simulink model "Appl_VentAdj_CtrlModel"  (R2018b)
settings: configuration reference "CodeConfig_10_ms" (kept outside this file)
undefined symbols (not defined in the file): D_VENT_LVL_1_PRECENT, D_VENT_LVL_2_PRECENT, D_VENT_LVL_3_PRECENT, FALSE, TRUE
libraries: DareLib x72, simulink x1
(part 4 of 4)

== stateflow chart Appl_VentAdj_CtrlModel/LogicCtrl/LocalAdjustCtrl/VentLevelDeal/LevelAquireFunction4/LevelAquireFunction ==
  state LevelAquire
    (default) -> (junction 92)
    LevelAquire -> (junction 92)
    (junction 92) -> (junction 95) [order 1] : /*加热功能禁能
        | || OFF 电
        | || 发动机不在运行中*/
        | [enVentStopReason.EN_VENT_STOP_R_NONE != DisableSts ...
        | || FALSE == EnableCfg ...
        | || enPowerModeSts.EN_OFF == PowerMode ...
        | || TRUE != EngineSts]
    (junction 92) -> (junction 94) [order 2] : {StopFlag = FALSE;}
    (junction 95) -> (junction 93) : {Level = enVentLvlSts.EN_VENT_LVL_OFF;
        | StopFlag = TRUE;}
    (junction 93) -> (junction 94)
    (junction 94) -> (junction 101)
    (junction 101) -> (junction 21) [order 1] : [StopFlag == FALSE]
    (junction 21) -> (junction 23) [order 1] : [enProjectType.EN_PROJECT_P20 == CarTypeCfg]
    (junction 101) -> (junction 104) [order 2] : {Level = enVentLvlSts.EN_VENT_LVL_OFF;}
    (junction 21) -> (junction 48) [order 2]
    (junction 23) -> (junction 82)
    (junction 82) -> (junction 84) [order 1] : /* 一键开启 且为Hmi控制 */
        | [5 == CAN_Message && Type == 0]
    (junction 82) -> (junction 25) [order 2]
    (junction 84) -> (junction 86) : {Level = CAN_Lvl + 1;}
    (junction 25) -> (junction 27) [order 1] : [4 == CAN_Message]
    (junction 25) -> (junction 29) [order 2] : {TempMsg = CAN_Message + 7;}
    (junction 27) -> (junction 57) : {Level = enVentLvlSts.EN_VENT_LVL_OFF;}
    (junction 48) -> (junction 50) [order 1] : [1 != CAN_Message]
    (junction 48) -> (junction 55) [order 2] : {Level = enVentLvlSts.EN_VENT_LVL_OFF;}
    (junction 50) -> (junction 52) : {TempMsg = CAN_Message;}
    (junction 52) -> (junction 29)
    (junction 29) -> (junction 32) [order 1] : [7 < TempMsg && 11 > TempMsg]
    (junction 29) -> (junction 36) [order 2] : {Level = 0xFF;}
    (junction 32) -> (junction 34)
    (junction 34) -> (junction 38) [order 1] : [8 == TempMsg]
    (junction 34) -> (junction 40) [order 2]
    (junction 38) -> (junction 59) : {Level = enVentLvlSts.EN_VENT_LVL_1;}
    (junction 40) -> (junction 42) [order 1] : [9 == TempMsg]
    (junction 40) -> (junction 46) [order 2] : {Level = enVentLvlSts.EN_VENT_LVL_3;}
    (junction 42) -> (junction 44) : {Level = enVentLvlSts.EN_VENT_LVL_2;}
    (junction 55) -> (junction 104)
    (junction 36) -> (junction 55)
    (junction 46) -> (junction 36)
    (junction 44) -> (junction 46)
    (junction 59) -> (junction 44)
    (junction 57) -> (junction 59)
    (junction 86) -> (junction 57)
    (junction 104) -> (junction 75)
  data: EnableCfg input uint8; CarTypeCfg input Enum: enProjectType; PowerMode input Enum: enPowerModeSts; EngineSts input uint8; CAN_Message input uint8; DisableSts input Enum: enVentStopReason; Level output uint8; TempMsg local uint8; TRUE parameter; FALSE parameter; CAN_Lvl input uint8; Type input; StopFlag local boolean

== stateflow chart Appl_VentAdj_CtrlModel/UpDataInputInfo/InputSignalProcess/VentMessage/VentMessage/MsgConflictFunction2/Function ==
  state HMI_MessageDeal [parallel]
    settings: executionOrder=1
    state Default
      en:
      HMI_Flag = FALSE;
    state Valid
      en:
      HMI_Flag = TRUE;
    (default) -> HMI_MessageDeal.Default
    HMI_MessageDeal.Default -> HMI_MessageDeal.Valid : /*HMI通风报文有效0x0:Inactive；0x1:Level 1；1档;0x2:Level 2；2档;0x3:Level 3；3档；0x4:OFF: 0x05 OPEN*/
        | [enVentLvlSts.EN_VENT_LVL_1 == HMI_Message ...
        | || enVentLvlSts.EN_VENT_LVL_2 == HMI_Message ...
        | || enVentLvlSts.EN_VENT_LVL_3 == HMI_Message ...
        | || 4 == HMI_Message || 5 == HMI_Message]
    HMI_MessageDeal.Valid -> HMI_MessageDeal.Default : /*HMI通风报文无效，20240507NXM增加关闭4*/
        | [enVentLvlSts.EN_VENT_LVL_1 != HMI_Message ...
        | && enVentLvlSts.EN_VENT_LVL_2 != HMI_Message ...
        | && enVentLvlSts.EN_VENT_LVL_3 != HMI_Message ...
        | && 4 != HMI_Message && 5 != HMI_Message]
  state Tbox_MessageDeal [parallel]
    settings: executionOrder=2
    state Default
      en:
      Tbox_Flag = FALSE;
    state Valid
      en:
      Tbox_Flag = TRUE;
    (default) -> Tbox_MessageDeal.Default
    Tbox_MessageDeal.Default -> Tbox_MessageDeal.Valid : /*Tbox通风报文有效0x0:No Request；0x1:Heat_1；0x2:Heat_2；0x3:Heat_3；0x4:Close*/
        | [enVentLvlSts.EN_VENT_LVL_1 == Tbox_Message ...
        | || enVentLvlSts.EN_VENT_LVL_2 == Tbox_Message ...
        | || enVentLvlSts.EN_VENT_LVL_3 == Tbox_Message ...
        | || 4 == Tbox_Message]
    Tbox_MessageDeal.Valid -> Tbox_MessageDeal.Default : /*Tbox通风报文无效，20240507NXM增加关闭4*/
        | [enVentLvlSts.EN_VENT_LVL_1 != Tbox_Message ...
        | && enVentLvlSts.EN_VENT_LVL_2 != Tbox_Message ...
        | && enVentLvlSts.EN_VENT_LVL_3 != Tbox_Message ...
        | && 4 != Tbox_Message]
  state MessageConflictDeal [parallel]
    settings: executionOrder=3
    state Default
      en,du:
      OutMsgHMI = HMI_Message;
      OutMsgTbox = Tbox_Message;
      MixConflictFlg = FALSE;
    state VentilateConflict
      en:
      OutMsgHMI = 0;
      OutMsgTbox = 0;
      MixConflictFlg = TRUE;
    state HeatConflict
      en:
      OutMsgHMI = 0;
      OutMsgTbox = 0;
      MixConflictFlg = FALSE;
    (default) -> MessageConflictDeal.Default
    MessageConflictDeal.Default -> VentilateConflict [order 2] : /*通风加热报文同时有效 且非关闭状态 */
        | [FALSE != VentValidFlag ...
        | && ((FALSE != HMI_Flag && 4 != HMI_Message) ...
        | || (FALSE != Tbox_Flag && 4 != Tbox_Message))]
    VentilateConflict -> MessageConflictDeal.Default [order 2] : /*通风加热报文不同时有效 或关闭，20240507NXM修改跳转顺序*/
        | [FALSE == VentValidFlag ...
        | || 4 == HMI_Message ...
        | || 4 == Tbox_Message]
    MessageConflictDeal.Default -> HeatConflict [order 1] : /*P20车型HMI、TBOX通风报文同时有效*/
        | [enProjectType.EN_PROJECT_P20 == CarTypeCfg ...
        | && FALSE != HMI_Flag ...
        | && FALSE != Tbox_Flag]
    HeatConflict -> MessageConflictDeal.Default [order 2] : /*非P20车型||P20车型通风报文不同时有效，20240507NXM*/
        | [enProjectType.EN_PROJECT_P20 != CarTypeCfg ...
        | || (enProjectType.EN_PROJECT_P20 == CarTypeCfg ...
        | && (FALSE == HMI_Flag || FALSE == Tbox_Flag))]
    VentilateConflict -> HeatConflict [order 1] : /*P20车型HMI、TBOX通风报文同时有效*/
        | [enProjectType.EN_PROJECT_P20 == CarTypeCfg ...
        | && FALSE != HMI_Flag ...
        | && FALSE != Tbox_Flag ...
        | && FALSE == VentValidFlag]
    HeatConflict -> VentilateConflict [order 1] : /*通风加热报文同时有效，20240507NXM*/
        | [FALSE != VentValidFlag ...
        | && (FALSE != HMI_Flag ...
        | || FALSE != Tbox_Flag)]
  data: CarTypeCfg input uint8; HMI_Message input; Tbox_Message input; VentValidFlag input uint8; FALSE parameter; OutMsgHMI output uint8; OutMsgTbox output uint8; HMI_Flag local uint8; Tbox_Flag local uint8; TRUE parameter; MixConflictFlg output uint8

== stateflow chart Appl_VentAdj_CtrlModel/LogicCtrl/LocalAdjustCtrl/VentLevelDeal/LevelAquireFunction5/LevelAquireFunction ==
  state LevelAquire
    (default) -> (junction 92)
    LevelAquire -> (junction 92)
    (junction 92) -> (junction 95) [order 1] : /*加热功能禁能
        | || OFF 电
        | || 发动机不在运行中*/
        | [enVentStopReason.EN_VENT_STOP_R_NONE != DisableSts ...
        | || FALSE == EnableCfg ...
        | || enPowerModeSts.EN_OFF == PowerMode ...
        | || TRUE != EngineSts]
    (junction 92) -> (junction 94) [order 2] : {StopFlag = FALSE;}
    (junction 95) -> (junction 93) : {Level = enVentLvlSts.EN_VENT_LVL_OFF;
        | StopFlag = TRUE;}
    (junction 93) -> (junction 94)
    (junction 94) -> (junction 101)
    (junction 101) -> (junction 21) [order 1] : [StopFlag == FALSE]
    (junction 21) -> (junction 23) [order 1] : [enProjectType.EN_PROJECT_P20 == CarTypeCfg]
    (junction 101) -> (junction 104) [order 2] : {Level = enVentLvlSts.EN_VENT_LVL_OFF;}
    (junction 21) -> (junction 48) [order 2]
    (junction 23) -> (junction 82)
    (junction 82) -> (junction 84) [order 1] : /* 一键开启 且为Hmi控制 */
        | [5 == CAN_Message && Type == 0]
    (junction 82) -> (junction 25) [order 2]
    (junction 84) -> (junction 86) : {Level = CAN_Lvl + 1;}
    (junction 25) -> (junction 27) [order 1] : [4 == CAN_Message]
    (junction 25) -> (junction 29) [order 2] : {TempMsg = CAN_Message + 7;}
    (junction 27) -> (junction 57) : {Level = enVentLvlSts.EN_VENT_LVL_OFF;}
    (junction 48) -> (junction 50) [order 1] : [1 != CAN_Message]
    (junction 48) -> (junction 55) [order 2] : {Level = enVentLvlSts.EN_VENT_LVL_OFF;}
    (junction 50) -> (junction 52) : {TempMsg = CAN_Message;}
    (junction 52) -> (junction 29)
    (junction 29) -> (junction 32) [order 1] : [7 < TempMsg && 11 > TempMsg]
    (junction 29) -> (junction 36) [order 2] : {Level = 0xFF;}
    (junction 32) -> (junction 34)
    (junction 34) -> (junction 38) [order 1] : [8 == TempMsg]
    (junction 34) -> (junction 40) [order 2]
    (junction 38) -> (junction 59) : {Level = enVentLvlSts.EN_VENT_LVL_1;}
    (junction 40) -> (junction 42) [order 1] : [9 == TempMsg]
    (junction 40) -> (junction 46) [order 2] : {Level = enVentLvlSts.EN_VENT_LVL_3;}
    (junction 42) -> (junction 44) : {Level = enVentLvlSts.EN_VENT_LVL_2;}
    (junction 55) -> (junction 104)
    (junction 36) -> (junction 55)
    (junction 46) -> (junction 36)
    (junction 44) -> (junction 46)
    (junction 59) -> (junction 44)
    (junction 57) -> (junction 59)
    (junction 86) -> (junction 57)
    (junction 104) -> (junction 75)
  data: EnableCfg input uint8; CarTypeCfg input Enum: enProjectType; PowerMode input Enum: enPowerModeSts; EngineSts input uint8; CAN_Message input uint8; DisableSts input Enum: enVentStopReason; Level output uint8; TempMsg local uint8; TRUE parameter; FALSE parameter; CAN_Lvl input uint8; Type input; StopFlag local boolean

== stateflow chart Appl_VentAdj_CtrlModel/UpDataInputInfo/InputSignalProcess/CommonPreconditionDeal/Deal ==
  state Default
    en:
    ComPCSatisfiedFlag = FALSE;
  state ValidSts
    en:
    ComPCSatisfiedFlag = TRUE;
  (default) -> Default
  Default -> ValidSts : /*(发动机运行中 || 整车运行状态满足) && 正常电压模式*/
      | [(TRUE == EngineRunningFlag || TRUE == VehicleRunFlag) ...
      | && enFinalPowerMode.EN_NORMAL_VOLT == VentAdj_VoltMode]
  ValidSts -> Default : /*(发动机不在运行中 && 整车运行状态不满足) || 非正常电压模式*/
      | [(TRUE != EngineRunningFlag && TRUE != VehicleRunFlag) ...
      | || enFinalPowerMode.EN_NORMAL_VOLT != VentAdj_VoltMode]
  data: EngineRunningFlag input; VehicleRunFlag input; ComPCSatisfiedFlag output uint8; TRUE parameter; FALSE parameter; VentAdj_VoltMode input

== stateflow chart Appl_VentAdj_CtrlModel/UpDataInputInfo/InputSignalProcess/VentMessage/VentMessage/MsgConflictFunction/Function ==
  state HMI_MessageDeal [parallel]
    settings: executionOrder=1
    state Default
      en:
      HMI_Flag = FALSE;
    state Valid
      en:
      HMI_Flag = TRUE;
    (default) -> HMI_MessageDeal.Default
    HMI_MessageDeal.Default -> HMI_MessageDeal.Valid : /*HMI通风报文有效0x0:Inactive；0x1:Level 1；1档;0x2:Level 2；2档;0x3:Level 3；3档；0x4:OFF: 0x05 OPEN*/
        | [enVentLvlSts.EN_VENT_LVL_1 == HMI_Message ...
        | || enVentLvlSts.EN_VENT_LVL_2 == HMI_Message ...
        | || enVentLvlSts.EN_VENT_LVL_3 == HMI_Message ...
        | || 4 == HMI_Message || 5 == HMI_Message]
    HMI_MessageDeal.Valid -> HMI_MessageDeal.Default : /*HMI通风报文无效，20240507NXM增加关闭4*/
        | [enVentLvlSts.EN_VENT_LVL_1 != HMI_Message ...
        | && enVentLvlSts.EN_VENT_LVL_2 != HMI_Message ...
        | && enVentLvlSts.EN_VENT_LVL_3 != HMI_Message ...
        | && 4 != HMI_Message && 5 != HMI_Message]
  state Tbox_MessageDeal [parallel]
    settings: executionOrder=2
    state Default
      en:
      Tbox_Flag = FALSE;
    state Valid
      en:
      Tbox_Flag = TRUE;
    (default) -> Tbox_MessageDeal.Default
    Tbox_MessageDeal.Default -> Tbox_MessageDeal.Valid : /*Tbox通风报文有效0x0:No Request；0x1:Heat_1；0x2:Heat_2；0x3:Heat_3；0x4:Close*/
        | [enVentLvlSts.EN_VENT_LVL_1 == Tbox_Message ...
        | || enVentLvlSts.EN_VENT_LVL_2 == Tbox_Message ...
        | || enVentLvlSts.EN_VENT_LVL_3 == Tbox_Message ...
        | || 4 == Tbox_Message]
    Tbox_MessageDeal.Valid -> Tbox_MessageDeal.Default : /*Tbox通风报文无效，20240507NXM增加关闭4*/
        | [enVentLvlSts.EN_VENT_LVL_1 != Tbox_Message ...
        | && enVentLvlSts.EN_VENT_LVL_2 != Tbox_Message ...
        | && enVentLvlSts.EN_VENT_LVL_3 != Tbox_Message ...
        | && 4 != Tbox_Message]
  state MessageConflictDeal [parallel]
    settings: executionOrder=3
    state Default
      en,du:
      OutMsgHMI = HMI_Message;
      OutMsgTbox = Tbox_Message;
      MixConflictFlg = FALSE;
    state VentilateConflict
      en:
      OutMsgHMI = 0;
      OutMsgTbox = 0;
      MixConflictFlg = TRUE;
    state HeatConflict
      en:
      OutMsgHMI = 0;
      OutMsgTbox = 0;
      MixConflictFlg = FALSE;
    (default) -> MessageConflictDeal.Default
    MessageConflictDeal.Default -> VentilateConflict [order 2] : /*通风加热报文同时有效 且非关闭状态 */
        | [FALSE != VentValidFlag ...
        | && ((FALSE != HMI_Flag && 4 != HMI_Message) ...
        | || (FALSE != Tbox_Flag && 4 != Tbox_Message))]
    VentilateConflict -> MessageConflictDeal.Default [order 2] : /*通风加热报文不同时有效 或关闭，20240507NXM修改跳转顺序*/
        | [FALSE == VentValidFlag ...
        | || 4 == HMI_Message ...
        | || 4 == Tbox_Message]
    MessageConflictDeal.Default -> HeatConflict [order 1] : /*P20车型HMI、TBOX通风报文同时有效*/
        | [enProjectType.EN_PROJECT_P20 == CarTypeCfg ...
        | && FALSE != HMI_Flag ...
        | && FALSE != Tbox_Flag]
    HeatConflict -> MessageConflictDeal.Default [order 2] : /*非P20车型||P20车型通风报文不同时有效，20240507NXM*/
        | [enProjectType.EN_PROJECT_P20 != CarTypeCfg ...
        | || (enProjectType.EN_PROJECT_P20 == CarTypeCfg ...
        | && (FALSE == HMI_Flag || FALSE == Tbox_Flag))]
    VentilateConflict -> HeatConflict [order 1] : /*P20车型HMI、TBOX通风报文同时有效*/
        | [enProjectType.EN_PROJECT_P20 == CarTypeCfg ...
        | && FALSE != HMI_Flag ...
        | && FALSE != Tbox_Flag ...
        | && FALSE == VentValidFlag]
    HeatConflict -> VentilateConflict [order 1] : /*通风加热报文同时有效，20240507NXM*/
        | [FALSE != VentValidFlag ...
        | && (FALSE != HMI_Flag ...
        | || FALSE != Tbox_Flag)]
  data: CarTypeCfg input uint8; HMI_Message input; Tbox_Message input; VentValidFlag input uint8; FALSE parameter; OutMsgHMI output uint8; OutMsgTbox output uint8; HMI_Flag local uint8; Tbox_Flag local uint8; TRUE parameter; MixConflictFlg output uint8
